simulink subsystem "mfc_F_est_cont"  (R2026a)
settings: Solver=VariableStepAuto
settings Model: Creator=devinbellll  LastModifiedBy=devinbellll

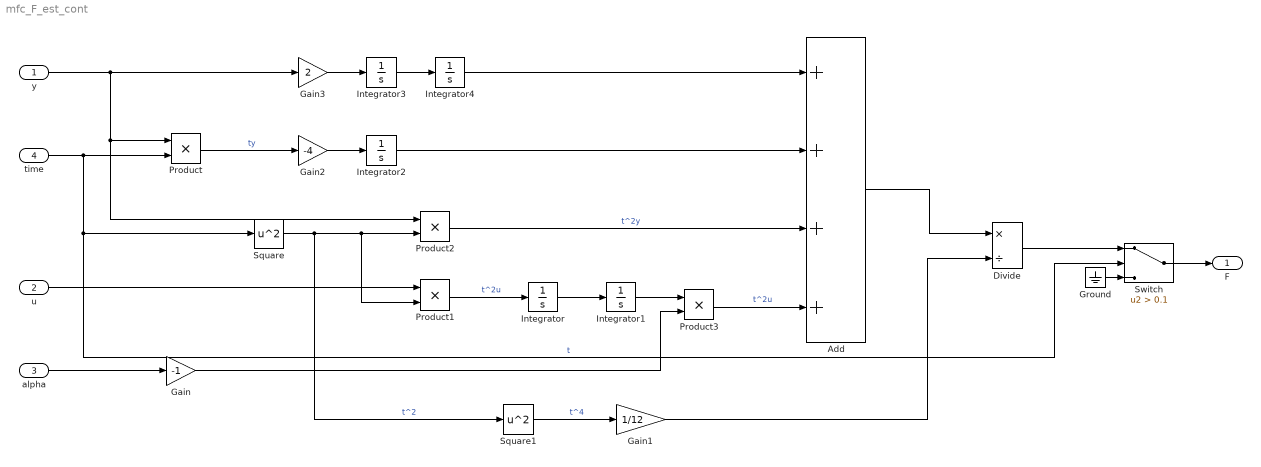
== system mfc_F_est_cont ==
  y : Inport
  u : Inport  Port=2
  alpha : Inport  Port=3
  time : Inport  Port=4
  Add : Sum  Inputs=++++
  Divide : Product  Inputs=*/
  Gain : Gain  Gain=-1
  Gain1 : Gain  Gain=1/12
  Gain2 : Gain  Gain=-4
  Gain3 : Gain  Gain=2
  Ground : Ground
  Integrator{,1..4} (5 alike) : Integrator
  Product{,1..3} (4 alike) : Product
  Square : Math  Operator=square
  Square1 : Math  Operator=square
  Switch : Switch  Criteria=u2 > Threshold  Threshold=0.1  SaturateOnIntegerOverflow=off  InputSameDT=off
  F : Outport
  wires:
  time/1 -> Product/2, Square/1, Switch/2  "t"
  y/1 -> Product/1, Product2/1, Gain3/1
  Square/1 -> Product1/2, Product2/2, Square1/1  "t^2"
  u/1 -> Product1/1
  Product/1 -> Gain2/1  "ty"
  Product1/1 -> Integrator/1  "t^2u"
  Product2/1 -> Add/3  "t^2y"
  Integrator/1 -> Integrator1/1
  Integrator1/1 -> Product3/1
  alpha/1 -> Gain/1
  Gain/1 -> Product3/2
  Product3/1 -> Add/4  "t^2u"
  Add/1 -> Divide/1
  Square1/1 -> Gain1/1  "t^4"
  Gain1/1 -> Divide/2
  Switch/1 -> F/1
  Ground/1 -> Switch/3
  Divide/1 -> Switch/1
  Gain2/1 -> Integrator2/1
  Integrator2/1 -> Add/2
  Gain3/1 -> Integrator3/1
  Integrator3/1 -> Integrator4/1
  Integrator4/1 -> Add/1
